simulink model "three_states_one_event_and_conditions"  (R2017b)
settings: Solver=FixedStepDiscrete  StartTime=0.0  StopTime=10.0  RelTol=1e-3
settings Model: Creator=flosch  LastModifiedBy=flosch
settings ConfigComp: CovScope=ReferencedModels  CovIncludeTopModel=off

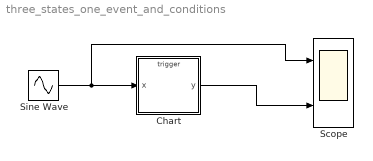
== system three_states_one_event_and_conditions ==
  Chart : Stateflow chart  TreatAsAtomicUnit=on
  Scope : Scope  NumInputPorts=2
  Sine Wave : Sin  SampleTime=0
  wires:
  Sine Wave/1 -> Scope/1, Chart/1(x)
  Chart/1(y) -> Scope/2

== stateflow chart three_states_one_event_and_conditions/Chart ==
  state Potato
    entry: y = x;
  state Kitten
    entry: y = 0;
  note: cyc = 7
      | obj = 6
      | lines = 7
  state Fish
    entry: y = 1;
  (default) -> Potato
  Potato -> Kitten [order 1] : Event_A [x <= 0]
  Potato -> Fish [order 2] : Event_A[x>0]
  data: t0 constant double =0.0; x input; y output
  events: Event_A input FUNCTION_CALL_EVENT
